simulink model "TST_FlSys_DetFlTnk"  (R2016b)
settings: Solver=FixedStepDiscrete  StartTime=0.0  StopTime=simTime  FixedStep=sampleTime  RelTol=1e-3
values from neighbouring files (symbols this model uses):
  testCase = 1    [initTST_FlSys_DetFlTnk_001.m]    (also in initTST_FlSys_DetFlTnk_002.m = 2)
libraries: simulink x3
settings Model: Creator=WF305  LastModifiedBy=WF305
settings DebuggingCC: SignalRangeChecking=error

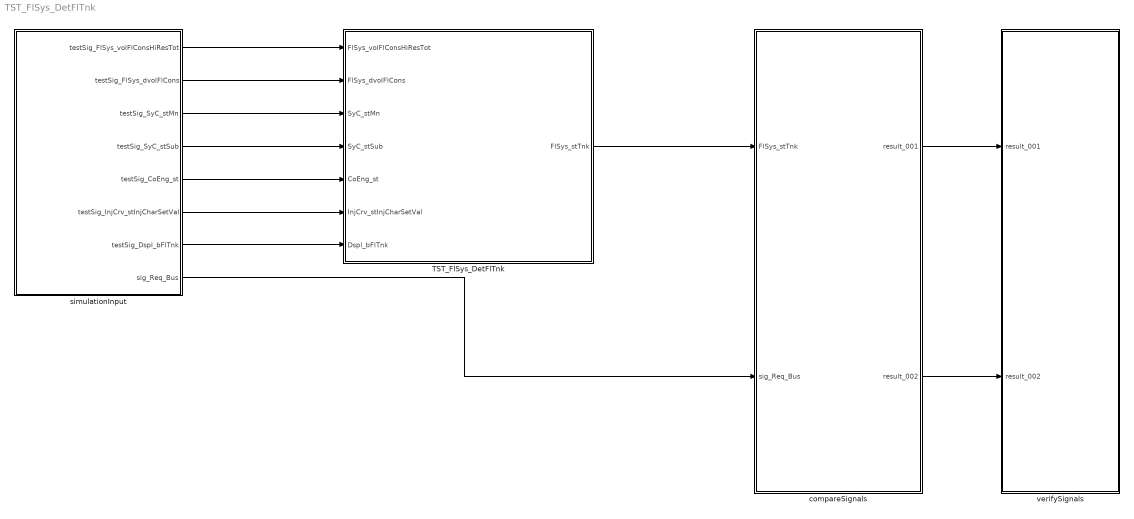
== system TST_FlSys_DetFlTnk ==
  TST_FlSys_DetFlTnk : Subsystem
  compareSignals : Subsystem
  simulationInput : Subsystem
  verifySignals : Subsystem
  wires:
  simulationInput/1(testSig_FlSys_volFlConsHiResTot) -> TST_FlSys_DetFlTnk/1(FlSys_volFlConsHiResTot)
  simulationInput/2(testSig_FlSys_dvolFlCons) -> TST_FlSys_DetFlTnk/2(FlSys_dvolFlCons)
  simulationInput/3(testSig_SyC_stMn) -> TST_FlSys_DetFlTnk/3(SyC_stMn)
  simulationInput/4(testSig_SyC_stSub) -> TST_FlSys_DetFlTnk/4(SyC_stSub)
  simulationInput/5(testSig_CoEng_st) -> TST_FlSys_DetFlTnk/5(CoEng_st)
  simulationInput/6(testSig_InjCrv_stInjCharSetVal) -> TST_FlSys_DetFlTnk/6(InjCrv_stInjCharSetVal)
  simulationInput/7(testSig_Dspl_bFlTnk) -> TST_FlSys_DetFlTnk/7(Dspl_bFlTnk)
  TST_FlSys_DetFlTnk/1(FlSys_stTnk) -> compareSignals/1(FlSys_stTnk)
  simulationInput/8(sig_Req_Bus) -> compareSignals/2(sig_Req_Bus)
  compareSignals/1(result_001) -> verifySignals/1(result_001)
  compareSignals/2(result_002) -> verifySignals/2(result_002)

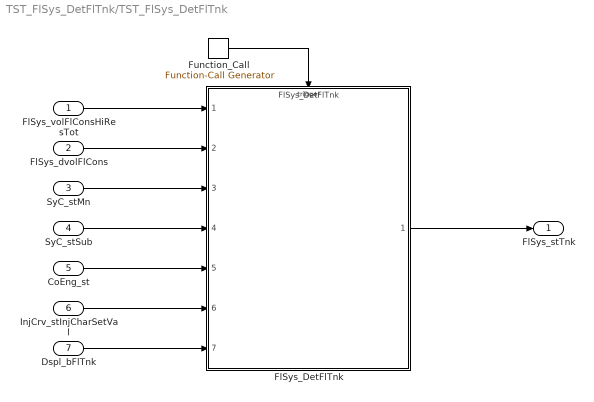
== system TST_FlSys_DetFlTnk/TST_FlSys_DetFlTnk ==
  FlSys_volFlConsHiResTot : Inport
  FlSys_dvolFlCons : Inport  Port=2
  SyC_stMn : Inport  Port=3
  SyC_stSub : Inport  Port=4
  CoEng_st : Inport  Port=5
  InjCrv_stInjCharSetVal : Inport  Port=6
  Dspl_bFlTnk : Inport  Port=7
  FlSys_DetFlTnk : ModelReference  ModelNameDialog=FlSys_DetFlTnk  ModelReferenceVersion=1.10  TriggerPortName=function  TriggerPortTriggerType=function-call  TriggerPortStatesWhenEnabling=held
  Function_Call : simulink/Ports & Subsystems/Function-Call Generator  sample_time=sampleTime  numberOfIterations=1
  FlSys_stTnk : Outport
  wires:
  Function_Call/1 -> FlSys_DetFlTnk/Trigger
  FlSys_volFlConsHiResTot/1 -> FlSys_DetFlTnk/1
  FlSys_dvolFlCons/1 -> FlSys_DetFlTnk/2
  SyC_stMn/1 -> FlSys_DetFlTnk/3
  SyC_stSub/1 -> FlSys_DetFlTnk/4
  CoEng_st/1 -> FlSys_DetFlTnk/5
  InjCrv_stInjCharSetVal/1 -> FlSys_DetFlTnk/6
  Dspl_bFlTnk/1 -> FlSys_DetFlTnk/7
  FlSys_DetFlTnk/1 -> FlSys_stTnk/1

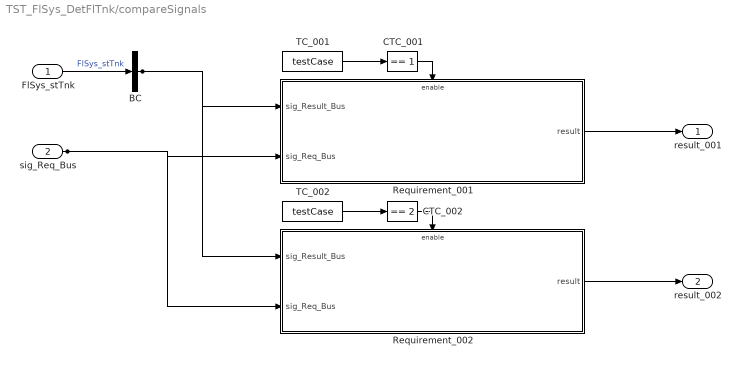
== system TST_FlSys_DetFlTnk/compareSignals ==
  FlSys_stTnk : Inport
  sig_Req_Bus : Inport  Port=2
  BC : BusCreator  Inputs=1
  CTC_001 : simulink/Logic and Bit Operations/Compare To Constant  relop===  const=1  OutDataTypeStr=boolean
  CTC_002 : simulink/Logic and Bit Operations/Compare To Constant  relop===  const=2  OutDataTypeStr=boolean
  Requirement_001 : Subsystem
  Requirement_002 : Subsystem
  TC_001 : Constant  Value=testCase
  TC_002 : Constant  Value=testCase
  result_001 : Outport
  result_002 : Outport  Port=2
  wires:
  FlSys_stTnk/1 -> BC/1  "FlSys_stTnk"
  TC_001/1 -> CTC_001/1
  CTC_001/1 -> Requirement_001/Enable
  sig_Req_Bus/1 -> Requirement_001/2(sig_Req_Bus), Requirement_002/2(sig_Req_Bus)
  BC/1 -> Requirement_001/1(sig_Result_Bus), Requirement_002/1(sig_Result_Bus)
  Requirement_001/1(result) -> result_001/1
  TC_002/1 -> CTC_002/1
  CTC_002/1 -> Requirement_002/Enable
  Requirement_002/1(result) -> result_002/1

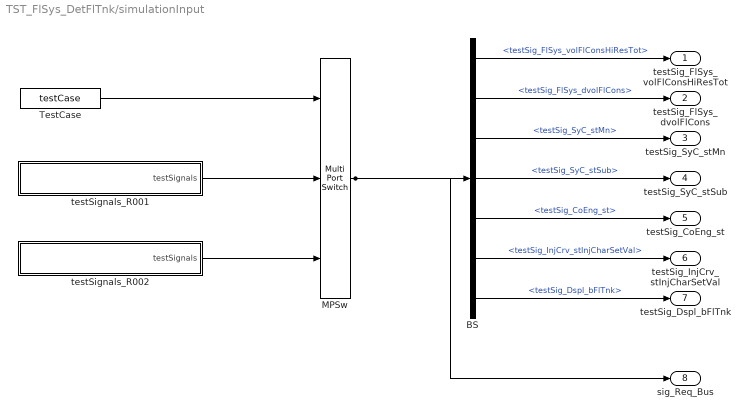
== system TST_FlSys_DetFlTnk/simulationInput ==
  BS : BusSelector  OutputSignals=testSig_FlSys_volFlConsHiResTot,testSig_FlSys_dvolFlCons,testSig_SyC_stMn,testSig_SyC_stSub,testSig_CoEng_st,testSig_InjCrv_stInjCharSetVal,testSig_Dspl_bFlTnk
  MPSw : MultiPortSwitch  Inputs=2  SaturateOnIntegerOverflow=on  InputSameDT=on
  TestCase : Constant  Value=testCase
  testSignals_R001 : Subsystem
  testSignals_R002 : Subsystem
  testSig_FlSys_volFlConsHiResTot : Outport
  testSig_FlSys_dvolFlCons : Outport  Port=2
  testSig_SyC_stMn : Outport  Port=3
  testSig_SyC_stSub : Outport  Port=4
  testSig_CoEng_st : Outport  Port=5
  testSig_InjCrv_stInjCharSetVal : Outport  Port=6
  testSig_Dspl_bFlTnk : Outport  Port=7
  sig_Req_Bus : Outport  Port=8
  wires:
  BS/1 -> testSig_FlSys_volFlConsHiResTot/1  "<testSig_FlSys_volFlConsHiResTot>"
  BS/2 -> testSig_FlSys_dvolFlCons/1  "<testSig_FlSys_dvolFlCons>"
  BS/3 -> testSig_SyC_stMn/1  "<testSig_SyC_stMn>"
  BS/4 -> testSig_SyC_stSub/1  "<testSig_SyC_stSub>"
  BS/5 -> testSig_CoEng_st/1  "<testSig_CoEng_st>"
  BS/6 -> testSig_InjCrv_stInjCharSetVal/1  "<testSig_InjCrv_stInjCharSetVal>"
  BS/7 -> testSig_Dspl_bFlTnk/1  "<testSig_Dspl_bFlTnk>"
  MPSw/1 -> BS/1, sig_Req_Bus/1
  TestCase/1 -> MPSw/1
  testSignals_R001/1(testSignals) -> MPSw/2
  testSignals_R002/1(testSignals) -> MPSw/3

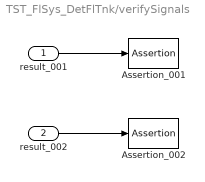
== system TST_FlSys_DetFlTnk/verifySignals ==
  result_001 : Inport
  result_002 : Inport  Port=2
  Assertion_001 : Assertion  Enabled=off
  Assertion_002 : Assertion  Enabled=off
  wires:
  result_001/1 -> Assertion_001/1
  result_002/1 -> Assertion_002/1

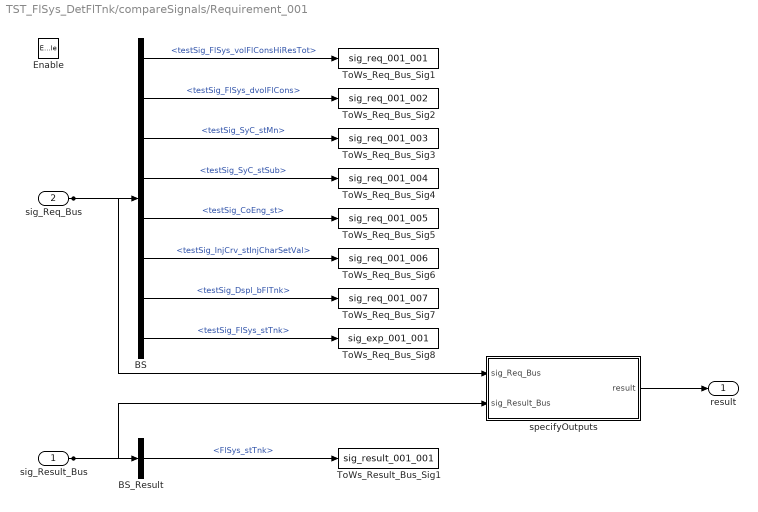
== system TST_FlSys_DetFlTnk/compareSignals/Requirement_001 ==
  sig_Result_Bus : Inport
  sig_Req_Bus : Inport  Port=2
  Enable : EnablePort
  BS : BusSelector  OutputSignals=testSig_FlSys_volFlConsHiResTot,testSig_FlSys_dvolFlCons,testSig_SyC_stMn,testSig_SyC_stSub,testSig_CoEng_st,testSig_InjCrv_stInjCharSetVal,testSig_Dspl_bFlTnk,testSig_FlSys_stTnk
  BS_Result : BusSelector  OutputSignals=FlSys_stTnk
  ToWs_Req_Bus_Sig1 : ToWorkspace  VariableName=sig_req_001_001  SaveFormat=Structure With Time
  ToWs_Req_Bus_Sig2 : ToWorkspace  VariableName=sig_req_001_002  SaveFormat=Structure With Time
  ToWs_Req_Bus_Sig3 : ToWorkspace  VariableName=sig_req_001_003  SaveFormat=Structure With Time
  ToWs_Req_Bus_Sig4 : ToWorkspace  VariableName=sig_req_001_004  SaveFormat=Structure With Time
  ToWs_Req_Bus_Sig5 : ToWorkspace  VariableName=sig_req_001_005  SaveFormat=Structure With Time
  ToWs_Req_Bus_Sig6 : ToWorkspace  VariableName=sig_req_001_006  SaveFormat=Structure With Time
  ToWs_Req_Bus_Sig7 : ToWorkspace  VariableName=sig_req_001_007  SaveFormat=Structure With Time
  ToWs_Req_Bus_Sig8 : ToWorkspace  VariableName=sig_exp_001_001  SaveFormat=Structure With Time
  ToWs_Result_Bus_Sig1 : ToWorkspace  VariableName=sig_result_001_001  SaveFormat=Structure With Time
  specifyOutputs : Subsystem
  result : Outport
  wires:
  sig_Req_Bus/1 -> BS/1, specifyOutputs/1(sig_Req_Bus)
  BS/1 -> ToWs_Req_Bus_Sig1/1  "<testSig_FlSys_volFlConsHiResTot>"
  BS/2 -> ToWs_Req_Bus_Sig2/1  "<testSig_FlSys_dvolFlCons>"
  BS/3 -> ToWs_Req_Bus_Sig3/1  "<testSig_SyC_stMn>"
  BS/4 -> ToWs_Req_Bus_Sig4/1  "<testSig_SyC_stSub>"
  BS/5 -> ToWs_Req_Bus_Sig5/1  "<testSig_CoEng_st>"
  BS/6 -> ToWs_Req_Bus_Sig6/1  "<testSig_InjCrv_stInjCharSetVal>"
  BS/7 -> ToWs_Req_Bus_Sig7/1  "<testSig_Dspl_bFlTnk>"
  BS/8 -> ToWs_Req_Bus_Sig8/1  "<testSig_FlSys_stTnk>"
  sig_Result_Bus/1 -> BS_Result/1, specifyOutputs/2(sig_Result_Bus)
  BS_Result/1 -> ToWs_Result_Bus_Sig1/1  "<FlSys_stTnk>"
  specifyOutputs/1(result) -> result/1

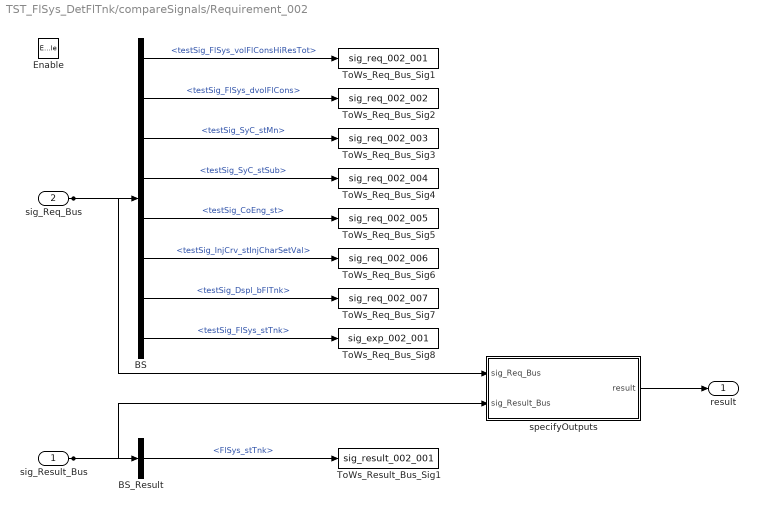
== system TST_FlSys_DetFlTnk/compareSignals/Requirement_002 ==
  sig_Result_Bus : Inport
  sig_Req_Bus : Inport  Port=2
  Enable : EnablePort
  BS : BusSelector  OutputSignals=testSig_FlSys_volFlConsHiResTot,testSig_FlSys_dvolFlCons,testSig_SyC_stMn,testSig_SyC_stSub,testSig_CoEng_st,testSig_InjCrv_stInjCharSetVal,testSig_Dspl_bFlTnk,testSig_FlSys_stTnk
  BS_Result : BusSelector  OutputSignals=FlSys_stTnk
  ToWs_Req_Bus_Sig1 : ToWorkspace  VariableName=sig_req_002_001  SaveFormat=Structure With Time
  ToWs_Req_Bus_Sig2 : ToWorkspace  VariableName=sig_req_002_002  SaveFormat=Structure With Time
  ToWs_Req_Bus_Sig3 : ToWorkspace  VariableName=sig_req_002_003  SaveFormat=Structure With Time
  ToWs_Req_Bus_Sig4 : ToWorkspace  VariableName=sig_req_002_004  SaveFormat=Structure With Time
  ToWs_Req_Bus_Sig5 : ToWorkspace  VariableName=sig_req_002_005  SaveFormat=Structure With Time
  ToWs_Req_Bus_Sig6 : ToWorkspace  VariableName=sig_req_002_006  SaveFormat=Structure With Time
  ToWs_Req_Bus_Sig7 : ToWorkspace  VariableName=sig_req_002_007  SaveFormat=Structure With Time
  ToWs_Req_Bus_Sig8 : ToWorkspace  VariableName=sig_exp_002_001  SaveFormat=Structure With Time
  ToWs_Result_Bus_Sig1 : ToWorkspace  VariableName=sig_result_002_001  SaveFormat=Structure With Time
  specifyOutputs : Subsystem
  result : Outport
  wires:
  sig_Req_Bus/1 -> BS/1, specifyOutputs/1(sig_Req_Bus)
  BS/1 -> ToWs_Req_Bus_Sig1/1  "<testSig_FlSys_volFlConsHiResTot>"
  BS/2 -> ToWs_Req_Bus_Sig2/1  "<testSig_FlSys_dvolFlCons>"
  BS/3 -> ToWs_Req_Bus_Sig3/1  "<testSig_SyC_stMn>"
  BS/4 -> ToWs_Req_Bus_Sig4/1  "<testSig_SyC_stSub>"
  BS/5 -> ToWs_Req_Bus_Sig5/1  "<testSig_CoEng_st>"
  BS/6 -> ToWs_Req_Bus_Sig6/1  "<testSig_InjCrv_stInjCharSetVal>"
  BS/7 -> ToWs_Req_Bus_Sig7/1  "<testSig_Dspl_bFlTnk>"
  BS/8 -> ToWs_Req_Bus_Sig8/1  "<testSig_FlSys_stTnk>"
  sig_Result_Bus/1 -> BS_Result/1, specifyOutputs/2(sig_Result_Bus)
  BS_Result/1 -> ToWs_Result_Bus_Sig1/1  "<FlSys_stTnk>"
  specifyOutputs/1(result) -> result/1

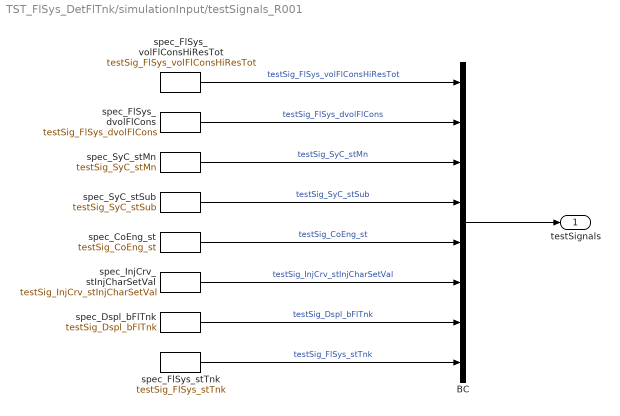
== system TST_FlSys_DetFlTnk/simulationInput/testSignals_R001 ==
  BC : BusCreator  Inputs=8
  spec_CoEng_st : FromWorkspace  VariableName=testSig_CoEng_st  Interpolate=off  OutputAfterFinalValue=Holding final value
  spec_Dspl_bFlTnk : FromWorkspace  VariableName=testSig_Dspl_bFlTnk  Interpolate=off  OutputAfterFinalValue=Holding final value
  spec_FlSys_dvolFlCons : FromWorkspace  VariableName=testSig_FlSys_dvolFlCons  Interpolate=off  OutputAfterFinalValue=Holding final value
  spec_FlSys_stTnk : FromWorkspace  VariableName=testSig_FlSys_stTnk  Interpolate=off  OutputAfterFinalValue=Holding final value
  spec_FlSys_volFlConsHiResTot : FromWorkspace  VariableName=testSig_FlSys_volFlConsHiResTot  Interpolate=off  OutputAfterFinalValue=Holding final value
  spec_InjCrv_stInjCharSetVal : FromWorkspace  VariableName=testSig_InjCrv_stInjCharSetVal  Interpolate=off  OutputAfterFinalValue=Holding final value
  spec_SyC_stMn : FromWorkspace  VariableName=testSig_SyC_stMn  Interpolate=off  OutputAfterFinalValue=Holding final value
  spec_SyC_stSub : FromWorkspace  VariableName=testSig_SyC_stSub  Interpolate=off  OutputAfterFinalValue=Holding final value
  testSignals : Outport
  wires:
  BC/1 -> testSignals/1
  spec_FlSys_volFlConsHiResTot/1 -> BC/1  "testSig_FlSys_volFlConsHiResTot"
  spec_FlSys_dvolFlCons/1 -> BC/2  "testSig_FlSys_dvolFlCons"
  spec_SyC_stMn/1 -> BC/3  "testSig_SyC_stMn"
  spec_SyC_stSub/1 -> BC/4  "testSig_SyC_stSub"
  spec_CoEng_st/1 -> BC/5  "testSig_CoEng_st"
  spec_InjCrv_stInjCharSetVal/1 -> BC/6  "testSig_InjCrv_stInjCharSetVal"
  spec_Dspl_bFlTnk/1 -> BC/7  "testSig_Dspl_bFlTnk"
  spec_FlSys_stTnk/1 -> BC/8  "testSig_FlSys_stTnk"

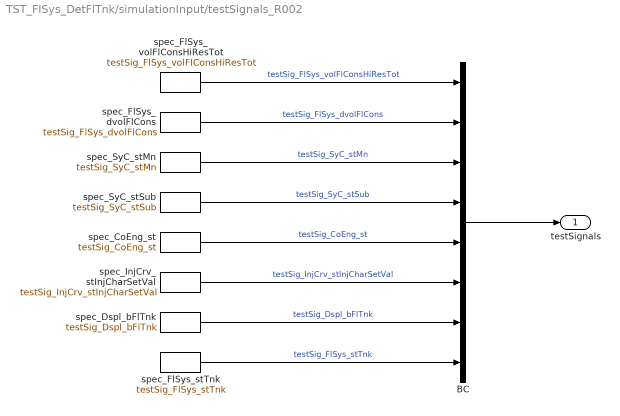
== system TST_FlSys_DetFlTnk/simulationInput/testSignals_R002 ==
  BC : BusCreator  Inputs=8
  spec_CoEng_st : FromWorkspace  VariableName=testSig_CoEng_st  Interpolate=off  OutputAfterFinalValue=Holding final value
  spec_Dspl_bFlTnk : FromWorkspace  VariableName=testSig_Dspl_bFlTnk  Interpolate=off  OutputAfterFinalValue=Holding final value
  spec_FlSys_dvolFlCons : FromWorkspace  VariableName=testSig_FlSys_dvolFlCons  Interpolate=off  OutputAfterFinalValue=Holding final value
  spec_FlSys_stTnk : FromWorkspace  VariableName=testSig_FlSys_stTnk  Interpolate=off  OutputAfterFinalValue=Holding final value
  spec_FlSys_volFlConsHiResTot : FromWorkspace  VariableName=testSig_FlSys_volFlConsHiResTot  Interpolate=off  OutputAfterFinalValue=Holding final value
  spec_InjCrv_stInjCharSetVal : FromWorkspace  VariableName=testSig_InjCrv_stInjCharSetVal  Interpolate=off  OutputAfterFinalValue=Holding final value
  spec_SyC_stMn : FromWorkspace  VariableName=testSig_SyC_stMn  Interpolate=off  OutputAfterFinalValue=Holding final value
  spec_SyC_stSub : FromWorkspace  VariableName=testSig_SyC_stSub  Interpolate=off  OutputAfterFinalValue=Holding final value
  testSignals : Outport
  wires:
  BC/1 -> testSignals/1
  spec_FlSys_volFlConsHiResTot/1 -> BC/1  "testSig_FlSys_volFlConsHiResTot"
  spec_FlSys_dvolFlCons/1 -> BC/2  "testSig_FlSys_dvolFlCons"
  spec_SyC_stMn/1 -> BC/3  "testSig_SyC_stMn"
  spec_SyC_stSub/1 -> BC/4  "testSig_SyC_stSub"
  spec_CoEng_st/1 -> BC/5  "testSig_CoEng_st"
  spec_InjCrv_stInjCharSetVal/1 -> BC/6  "testSig_InjCrv_stInjCharSetVal"
  spec_Dspl_bFlTnk/1 -> BC/7  "testSig_Dspl_bFlTnk"
  spec_FlSys_stTnk/1 -> BC/8  "testSig_FlSys_stTnk"

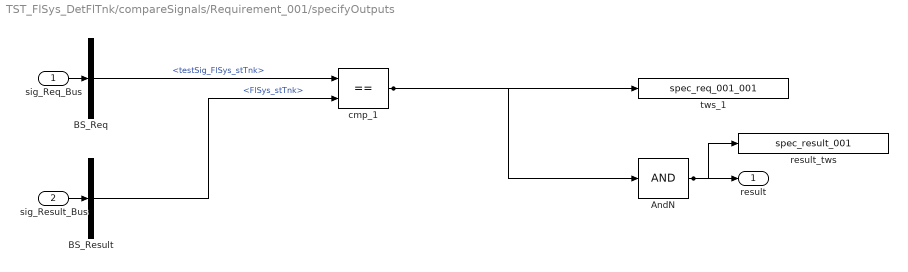
== system TST_FlSys_DetFlTnk/compareSignals/Requirement_001/specifyOutputs ==
  sig_Req_Bus : Inport
  sig_Result_Bus : Inport  Port=2
  AndN : Logic  Inputs=1
  BS_Req : BusSelector  OutputSignals=testSig_FlSys_stTnk
  BS_Result : BusSelector  OutputSignals=FlSys_stTnk
  cmp_1 : RelationalOperator  Operator===  RndMeth=Nearest  InputSameDT=on
  result_tws : ToWorkspace  VariableName=spec_result_001
  tws_1 : ToWorkspace  VariableName=spec_req_001_001
  result : Outport
  wires:
  sig_Req_Bus/1 -> BS_Req/1
  sig_Result_Bus/1 -> BS_Result/1
  AndN/1 -> result/1, result_tws/1
  BS_Req/1 -> cmp_1/1  "<testSig_FlSys_stTnk>"
  BS_Result/1 -> cmp_1/2  "<FlSys_stTnk>"
  cmp_1/1 -> tws_1/1, AndN/1

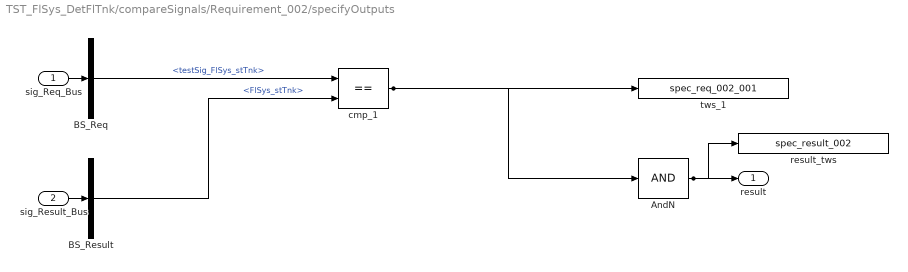
== system TST_FlSys_DetFlTnk/compareSignals/Requirement_002/specifyOutputs ==
  sig_Req_Bus : Inport
  sig_Result_Bus : Inport  Port=2
  AndN : Logic  Inputs=1
  BS_Req : BusSelector  OutputSignals=testSig_FlSys_stTnk
  BS_Result : BusSelector  OutputSignals=FlSys_stTnk
  cmp_1 : RelationalOperator  Operator===  RndMeth=Nearest  InputSameDT=on
  result_tws : ToWorkspace  VariableName=spec_result_002
  tws_1 : ToWorkspace  VariableName=spec_req_002_001
  result : Outport
  wires:
  sig_Req_Bus/1 -> BS_Req/1
  sig_Result_Bus/1 -> BS_Result/1
  AndN/1 -> result/1, result_tws/1
  BS_Req/1 -> cmp_1/1  "<testSig_FlSys_stTnk>"
  BS_Result/1 -> cmp_1/2  "<FlSys_stTnk>"
  cmp_1/1 -> tws_1/1, AndN/1
